simulink model "ECS_FOS"  (R2013b)
settings: Solver=ode45  StartTime=0.0  StopTime=10.0  RelTol=1e-3
values from neighbouring files (symbols this model uses):
  FuelBurn = [0 0 0 0 0 0 0 0 0 0 0 0 ... (18249 elements, 1x18249)]    [Benchmark_data1.mat]
undefined symbols (not defined in the file or in its folder): F1, F2, HUGHES_TREITLER, PN_70147
libraries: PowerFlowLib x47, simulink x6
(part 1 of 2)
settings Model: Creator=mwillms4  LastModifiedBy=mwillms4

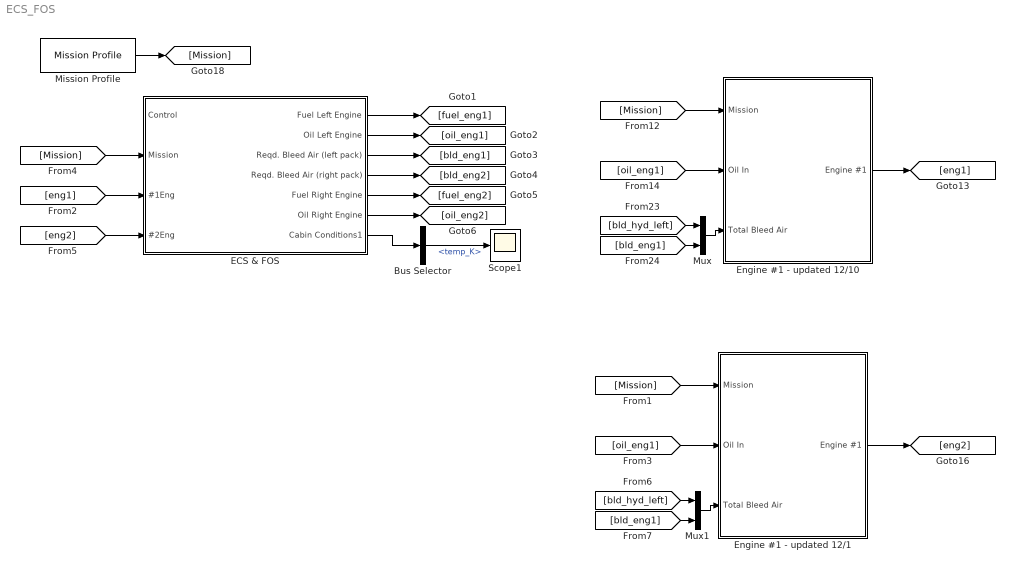
== system ECS_FOS ==
  Bus Selector : BusSelector  OutputSignals=temp_K
  "ECS & FOS " : Subsystem
  Engine #1 - updated 12/1 : Subsystem
  Engine #1 - updated 12/10 : Subsystem
  Mission Profile : PowerFlowLib/Mission Profile/Mission Profile  mssn_check=off  mssn_prof=MSSN  del_P=0  del_T=0  del_rho=0  pres_msl=101.3  temp_msl=15  dens_msl=1.229
  Mux : Mux  Inputs=2
  Mux1 : Mux  Inputs=2
  Scope1 : Scope
      settings: YMin=290  YMax=300
  wires:
  Mission Profile/1 -> [Mission]
  [eng1] -> "ECS & FOS "/3(#1Eng)
  [Mission] -> "ECS & FOS "/2(Mission)
  [eng2] -> "ECS & FOS "/4(#2Eng)
  Engine #1 - updated 12/10/1(Engine #1) -> [eng1]
  Engine #1 - updated 12/1/1(Engine #1) -> [eng2]
  [Mission] -> Engine #1 - updated 12/10/1(Mission)
  [oil_eng1] -> Engine #1 - updated 12/10/2(Oil In)
  Mux/1 -> Engine #1 - updated 12/10/3(Total Bleed Air)
  [bld_eng1] -> Mux/2
  [bld_hyd_left] -> Mux/1
  Bus Selector/1 -> Scope1/1  "<temp_K>"
  "ECS & FOS "/1("Fuel Left Engine ") -> [fuel_eng1]
  "ECS & FOS "/2(Oil Left Engine) -> [oil_eng1]
  "ECS & FOS "/3(Reqd. Bleed Air (left pack)) -> [bld_eng1]
  "ECS & FOS "/4(Reqd. Bleed Air (right pack)) -> [bld_eng2]
  "ECS & FOS "/5(Fuel Right Engine) -> [fuel_eng2]
  "ECS & FOS "/6(Oil Right Engine) -> [oil_eng2]
  "ECS & FOS "/7(Cabin Conditions1) -> Bus Selector/1
  [Mission] -> Engine #1 - updated 12/1/1(Mission)
  [oil_eng1] -> Engine #1 - updated 12/1/2(Oil In)
  Mux1/1 -> Engine #1 - updated 12/1/3(Total Bleed Air)
  [bld_eng1] -> Mux1/2
  [bld_hyd_left] -> Mux1/1

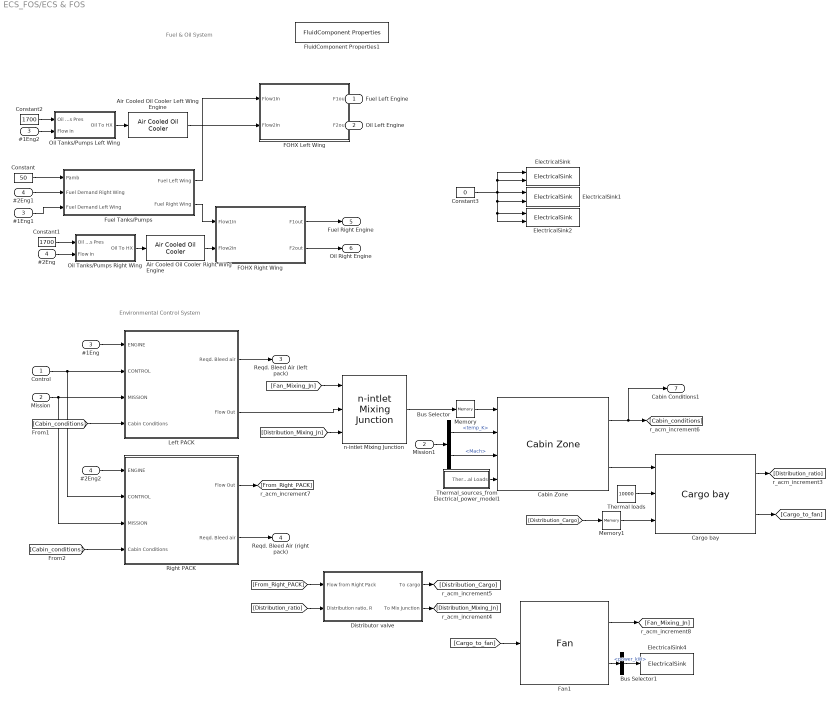
== system ECS_FOS/ECS & FOS  ==
  note: Fuel & Oil System
  note: Environmental Control System
  Control : Inport
  Mission : Inport  Port=2
  #1Eng : Inport  Port=3
  #2Eng : Inport  Port=4
  #1Eng1 : InportShadow  Port=3
  #1Eng2 : InportShadow  Port=3
  #2Eng1 : InportShadow  Port=4
  #2Eng2 : InportShadow  Port=4
  Air Cooled Oil Cooler Left Wing Engine : PowerFlowLib/Energy & Power Systems/Thermal/Oil/Air Cooled Oil Cooler  fileslct=off  filename=HeatExchangers.mat  filedir=C:\Users\mwillms4\Dropbox\School\Graduate\Research\PowerFlow Summer 2013\PropertyTables\HeatExchangers.mat  refresh=off  hx=HUGHES_TREITLER - PN_70147  bypass_full=1  bypass_none=100  hx_delP=82.74  hx_P=2068  hx_Qdot=24.27  hx_Vdot=0.000505  hx_mass=4.42
  Air Cooled Oil Cooler Right Wing Engine : PowerFlowLib/Energy & Power Systems/Thermal/Oil/Air Cooled Oil Cooler  fileslct=off  filename=HeatExchangers.mat  filedir=C:\Users\mwillms4\Dropbox\School\Graduate\Research\PowerFlow Summer 2013\PropertyTables\HeatExchangers.mat  refresh=off  hx=HUGHES_TREITLER - PN_70147  bypass_full=1  bypass_none=100  hx_delP=82.74  hx_P=2068  hx_Qdot=24.27  hx_Vdot=0.000505  hx_mass=4.42
  Bus Selector : BusSelector  OutputSignals=Flight parameters.temp_K,Flight parameters.Mach
  Bus Selector1 : BusSelector  OutputSignals=power_kW
  Cabin Zone : PowerFlowLib/Energy & Power Systems/Thermal/ECS/Cabin Zone  A_fuselage=320  V_cab=130.3  n_pass=176  L_shell=0.003  K_shell=1  L_insulation=0.02  K_insulation=1  L_coating=0.002  K_coating=1  Vdot_sa_pass=0.009438  q_pass=60  RAR=.25  h_outside=1  h_inside=1
  Cargo bay : PowerFlowLib/Energy & Power Systems/Thermal/ECS/Cargo bay  T_cargo_K=305
  Constant : Constant  Value=50
  Constant1 : Constant  Value=1700
  Constant2 : Constant  Value=1700
  Constant3 : Constant  Value=0
  Distributor valve : Subsystem
  ElectricalSink : PowerFlowLib/Support Functions//Tools/ElectricalSink  Tag=Flow  Description=TwoPhase  load_loc=Empennage  ACDC_load=AC  units=Kilowatts  unq_id=9254
  ElectricalSink1 : PowerFlowLib/Support Functions//Tools/ElectricalSink  Tag=Flow  Description=TwoPhase  load_loc=Cagobay  ACDC_load=AC  units=Kilowatts  unq_id=3572
  ElectricalSink2 : PowerFlowLib/Support Functions//Tools/ElectricalSink  Tag=Flow  Description=TwoPhase  load_loc=Cabin  ACDC_load=AC  units=Kilowatts  unq_id=7814
  ElectricalSink4 : PowerFlowLib/Support Functions//Tools/ElectricalSink  Tag=Flow  Description=TwoPhase  load_loc=Cabin  ACDC_load=DC  units=Kilowatts  unq_id=7783
  FOHX Left Wing : Subsystem  Description=TwoPhase  mask{fld1=JP8, fld2=LubeOil7808, alpha1=80, alpha2=80, N1=10, N2=10, A1_c=.1, A2_c=.1, A1_s=.25, A2_s=.25, P1init=620.5, P2init=620.5}
      mask prompts: fld1 "Fluid 1 Type"; fld2 "Fluid 2 Type"; alpha1 "Fluid 1 HTC [W/m² K]"; alpha2 "Fluid 2 HTC [W/m² K]"; N1 "Flow 1: Number of Channels"; N2 "Flow 2: Number of Channels"; A1_c "Flow 1: Cross-sectional area [m^2]"; A2_c "Flow 2: Cross-sectional area [m^2]"; A1_s "Flow 1: Total surface area [m^2]"; A2_s "Flow 2: Total surface area [m^2]"; P1init "Flow 1 Pressure [kPa]"; P2init "Flow 2 Pressure [kPa]"
      mask init:
      | %load TMSFluidProperties
      | %eval(['SF = FluidProp.SinglePhase.' get_param(gcb,'fld_type1') ';']);
      | %eval(['F = FluidProp.TwoPhase.' get_param(gcb,'fld_type2') ';']);
      | %FluidProp = FluidProp.TwoPhase.R134a; 
      | %{
      | if strcmp(get_param(bdroot,'SimulationStatus'),'initializing') ;
      |     load TwoPhaseProp_Evap
      |     TwoPhaseProp = TwoPhaseProp_Evap;
      |     Evaporator_Init_AFRL;
      | end
      | TMS_SetPhysSigs
      | if strcmp(get_param(gcb,'fld_type1'),'MoistAir')
      |     notair = 0 ; 
      | else
      |     notair = 1 ;
      | end
      | %}
      mask TypeOptions fld1: JP8
      mask TypeOptions fld2: LubeOil7808
      mask Display:
      | port_label('input',1,'Fuel In','TexMode','on') ;
      | port_label('input',2,'Oil In','TexMode','on') ;
      | port_label('output',1,'Fuel Out','TexMode','on') ;
      | port_label('output',2,'Oil Out','TexMode','on') ;
  FOHX Right Wing : Subsystem  Description=TwoPhase  mask{fld1=JP8, fld2=LubeOil7808, alpha1=80, alpha2=80, N1=10, N2=10, A1_c=.1, A2_c=.1, A1_s=.25, A2_s=.25, P1init=620.5, P2init=620.5}
      mask prompts: fld1 "Fluid 1 Type"; fld2 "Fluid 2 Type"; alpha1 "Fluid 1 HTC [W/m² K]"; alpha2 "Fluid 2 HTC [W/m² K]"; N1 "Flow 1: Number of Channels"; N2 "Flow 2: Number of Channels"; A1_c "Flow 1: Cross-sectional area [m^2]"; A2_c "Flow 2: Cross-sectional area [m^2]"; A1_s "Flow 1: Total surface area [m^2]"; A2_s "Flow 2: Total surface area [m^2]"; P1init "Flow 1 Pressure [kPa]"; P2init "Flow 2 Pressure [kPa]"
      mask init: same as ECS_FOS/ECS & FOS /FOHX Left Wing
      mask TypeOptions fld1: JP8
      mask TypeOptions fld2: LubeOil7808
      mask Display:
      | port_label('input',1,'Fuel In','TexMode','on') ;
      | port_label('input',2,'Oil In','TexMode','on') ;
      | port_label('output',1,'Fuel Out','TexMode','on') ;
      | port_label('output',2,'Oil Out','TexMode','on') ;
  Fan1 : PowerFlowLib/Energy & Power Systems/Thermal/ECS/Fan  N_fan=1725
  FluidComponent Properties1 : PowerFlowLib/Support Functions//Tools/FluidComponent Properties  fuelprop=FluidProp_JetA3638.mat  oilprop=OilProp.mat  airprop=AirProp.mat  pumpprop=PumpProp.mat  fanprop=Fanmap.mat  compprop=CompProp.mat  heatexprop=HeatExchangers.mat
  Fuel Tanks/Pumps : Subsystem
  Left PACK : Subsystem
  Memory : Memory
  Memory1 : Memory
  Mission1 : InportShadow  Port=2
  Oil Tanks/Pumps Left Wing : Subsystem
  Oil Tanks/Pumps Right Wing : Subsystem
  Right PACK : Subsystem
  Thermal loads : Constant  Value=10000
  Thermal_sources_from Electrical_power_model1 : Subsystem
  n-intlet Mixing Junction : PowerFlowLib/Energy & Power Systems/Thermal/ECS/n-intlet Mixing Junction  no_inlets=3  d_in_1=0.1  d_in_2=0.1  d_out=0.2
  "Fuel Left Engine " : Outport
  Oil Left Engine : Outport  Port=2
  Reqd. Bleed Air (left pack) : Outport  Port=3
  Reqd. Bleed Air (right pack) : Outport  Port=4
  Fuel Right Engine : Outport  Port=5
  Oil Right Engine : Outport  Port=6
  Cabin Conditions1 : Outport  Port=7
  wires:
  Cargo bay/2 -> [Cargo_to_fan]
  Cabin Zone/2 -> Cargo bay/1
  Memory1/1 -> Cargo bay/3
  Thermal loads/1 -> Cargo bay/2
  Cargo bay/1 -> [Distribution_ratio]
  [Distribution_Cargo] -> Memory1/1
  Fan1/2 -> Bus Selector1/1
  Fan1/1 -> [Fan_Mixing_Jn]
  [Cargo_to_fan] -> Fan1/1
  Bus Selector1/1 -> ElectricalSink4/1  "<power_kW>"
  [Distribution_Mixing_Jn] -> n-intlet Mixing Junction/3
  Right PACK/1(Flow Out) -> [From_Right_PACK]
  [Cabin_conditions] -> Left PACK/4(Cabin Conditions)
  [Cabin_conditions] -> Right PACK/4(Cabin Conditions)
  [Fan_Mixing_Jn] -> n-intlet Mixing Junction/1
  Cabin Zone/1 -> [Cabin_conditions], Cabin Conditions1/1
  Distributor valve/1(To cargo) -> [Distribution_Cargo]
  Distributor valve/2(To Mix Junction) -> [Distribution_Mixing_Jn]
  [From_Right_PACK] -> Distributor valve/1(Flow from Right Pack)
  [Distribution_ratio] -> Distributor valve/2("Distribution ratio, R")
  #2Eng2/1 -> Right PACK/1(ENGINE)
  #1Eng/1 -> Left PACK/1(ENGINE)
  #2Eng/1 -> Oil Tanks/Pumps Right Wing/2(Flow In)
  #1Eng1/1 -> Fuel Tanks/Pumps/3(Fuel Demand Left Wing)
  #2Eng1/1 -> Fuel Tanks/Pumps/2(Fuel Demand Right Wing)
  #1Eng2/1 -> Oil Tanks/Pumps Left Wing/2(Flow In)
  Memory/1 -> Cabin Zone/1
  Left PACK/2(Flow Out) -> n-intlet Mixing Junction/2
  Thermal_sources_from Electrical_power_model1/1(Thermal Loads) -> Cabin Zone/4
  Bus Selector/2 -> Cabin Zone/3  "<Mach>"
  Bus Selector/1 -> Cabin Zone/2  "<temp_K>"
  Mission1/1 -> Bus Selector/1
  n-intlet Mixing Junction/1 -> Memory/1
  Constant3/1 -> ElectricalSink/2, ElectricalSink/1, ElectricalSink1/2, ElectricalSink2/2, ElectricalSink2/1, ElectricalSink1/1
  FOHX Left Wing/2(F2out) -> Oil Left Engine/1
  FOHX Right Wing/2(F2out) -> Oil Right Engine/1
  FOHX Left Wing/1(F1out) -> "Fuel Left Engine "/1
  Fuel Tanks/Pumps/1(Fuel Left Wing) -> FOHX Left Wing/1(Flow1In)
  Constant2/1 -> Oil Tanks/Pumps Left Wing/1(Oil Sys Pres)
  Oil Tanks/Pumps Left Wing/1(Oil To HX) -> Air Cooled Oil Cooler Left Wing Engine/1
  Air Cooled Oil Cooler Left Wing Engine/1 -> FOHX Left Wing/2(Flow2In)
  FOHX Right Wing/1(F1out) -> Fuel Right Engine/1
  Constant1/1 -> Oil Tanks/Pumps Right Wing/1(Oil Sys Pres)
  Oil Tanks/Pumps Right Wing/1(Oil To HX) -> Air Cooled Oil Cooler Right Wing Engine/1
  Fuel Tanks/Pumps/2(Fuel Right Wing) -> FOHX Right Wing/1(Flow1In)
  Air Cooled Oil Cooler Right Wing Engine/1 -> FOHX Right Wing/2(Flow2In)
  Constant/1 -> Fuel Tanks/Pumps/1(Pamb)
  Right PACK/2(Reqd. Bleed air) -> Reqd. Bleed Air (right pack)/1
  Mission/1 -> Right PACK/3(MISSION), Left PACK/3(MISSION)
  Control/1 -> Right PACK/2(CONTROL), Left PACK/2(CONTROL)
  Left PACK/1(Reqd. Bleed air) -> Reqd. Bleed Air (left pack)/1

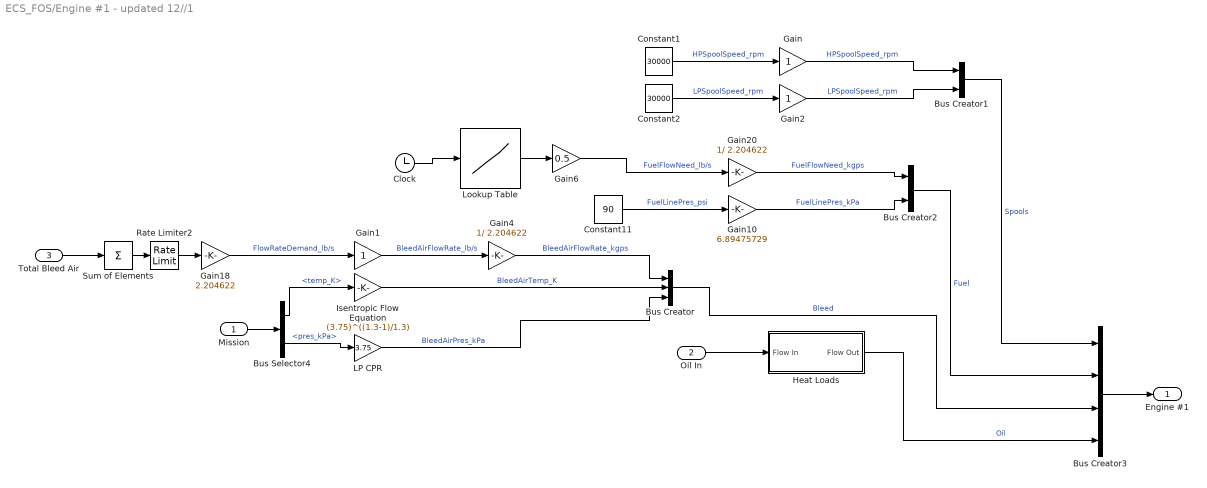
== system ECS_FOS/Engine #1 - updated 12//1 ==
  Mission : Inport
  Oil In : Inport  Port=2
  Total Bleed Air : Inport  Port=3
  Bus Creator : BusCreator  Inputs=3
  Bus Creator1 : BusCreator  Inputs=2
  Bus Creator2 : BusCreator  Inputs=2
  Bus Creator3 : BusCreator
  Bus Selector4 : BusSelector  OutputSignals=Flight parameters.temp_K,Flight parameters.pres_kPa
  Clock : Clock
  Constant1 : Constant  Value=30000
  Constant11 : Constant  Value=90
  Constant2 : Constant  Value=30000
  Gain : Gain
  Gain1 : Gain
  Gain10 : Gain  Gain=6.89475729
  Gain18 : Gain  Gain=2.204622
  Gain2 : Gain
  Gain20 : Gain  Gain=1/ 2.204622
  Gain4 : Gain  Gain=1/ 2.204622
  Gain6 : Gain  Gain=0.5
  Heat Loads : Subsystem
  Isentropic Flow Equation : Gain  Gain=(3.75)^((1.3-1)/1.3)
  LP CPR : Gain  Gain=3.75
  Lookup Table : Lookup  InputValues=[0:size(FuelBurn,2)-1]  Table=FuelBurn
  Rate Limiter2 : RateLimiter
  Sum of Elements : Sum  Inputs=+
  Engine #1 : Outport
  wires:
  Bus Creator3/1 -> Engine #1/1
  Lookup Table/1 -> Gain6/1
  Clock/1 -> Lookup Table/1
  Bus Selector4/1 -> Isentropic Flow Equation/1  "<temp_K>"
  Bus Selector4/2 -> LP CPR/1  "<pres_kPa>"
  Mission/1 -> Bus Selector4/1
  Sum of Elements/1 -> Rate Limiter2/1
  Bus Creator2/1 -> Bus Creator3/2  "Fuel"
  Bus Creator1/1 -> Bus Creator3/1  "Spools"
  Bus Creator/1 -> Bus Creator3/3  "Bleed"
  Heat Loads/1(Flow Out) -> Bus Creator3/4  "Oil"
  Oil In/1 -> Heat Loads/1(Flow In)
  Rate Limiter2/1 -> Gain18/1
  Gain18/1 -> Gain1/1  "FlowRateDemand_lb/s"
  Total Bleed Air/1 -> Sum of Elements/1
  Gain/1 -> Bus Creator1/1  "HPSpoolSpeed_rpm"
  Constant1/1 -> Gain/1  "HPSpoolSpeed_rpm"
  Gain2/1 -> Bus Creator1/2  "LPSpoolSpeed_rpm"
  Constant2/1 -> Gain2/1  "LPSpoolSpeed_rpm"
  Gain4/1 -> Bus Creator/1  "BleedAirFlowRate_kgps"
  Gain1/1 -> Gain4/1  "BleedAirFlowRate_lb/s"
  Isentropic Flow Equation/1 -> Bus Creator/2  "BleedAirTemp_K"
  LP CPR/1 -> Bus Creator/3  "BleedAirPres_kPa"
  Gain20/1 -> Bus Creator2/1  "FuelFlowNeed_kgps"
  Gain6/1 -> Gain20/1  "FuelFlowNeed_lb/s"
  Gain10/1 -> Bus Creator2/2  "FuelLinePres_kPa"
  Constant11/1 -> Gain10/1  "FuelLinePres_psi"

== system ECS_FOS/Engine #1 - updated 12//10 ==
  Mission : Inport
  Oil In : Inport  Port=2
  Total Bleed Air : Inport  Port=3
  Bus Creator : BusCreator  Inputs=3
  Bus Creator1 : BusCreator  Inputs=2
  Bus Creator2 : BusCreator  Inputs=2
  Bus Creator3 : BusCreator
  Bus Selector4 : BusSelector  OutputSignals=Flight parameters.temp_K,Flight parameters.pres_kPa
  Clock : Clock
  Constant1 : Constant  Value=30000
  Constant11 : Constant  Value=90
  Constant2 : Constant  Value=30000
  Gain : Gain
  Gain1 : Gain
  Gain10 : Gain  Gain=6.89475729
  Gain18 : Gain  Gain=2.204622
  Gain2 : Gain
  Gain20 : Gain  Gain=1/ 2.204622
  Gain4 : Gain  Gain=1/ 2.204622
  Gain6 : Gain  Gain=0.5
  Heat Loads : Subsystem
  Isentropic Flow Equation : Gain  Gain=(3.75)^((1.3-1)/1.3)
  LP CPR : Gain  Gain=3.75
  Lookup Table : Lookup  InputValues=[0:size(FuelBurn,2)-1]  Table=FuelBurn
  Rate Limiter2 : RateLimiter
  Sum of Elements : Sum  Inputs=+
  Engine #1 : Outport
  wires:
  Constant11/1 -> Gain10/1  "FuelLinePres_psi"
  Gain10/1 -> Bus Creator2/2  "FuelLinePres_kPa"
  Gain6/1 -> Gain20/1  "FuelFlowNeed_lb/s"
  Gain20/1 -> Bus Creator2/1  "FuelFlowNeed_kgps"
  LP CPR/1 -> Bus Creator/3  "BleedAirPres_kPa"
  Isentropic Flow Equation/1 -> Bus Creator/2  "BleedAirTemp_K"
  Gain1/1 -> Gain4/1  "BleedAirFlowRate_lb/s"
  Gain4/1 -> Bus Creator/1  "BleedAirFlowRate_kgps"
  Constant2/1 -> Gain2/1  "LPSpoolSpeed_rpm"
  Gain2/1 -> Bus Creator1/2  "LPSpoolSpeed_rpm"
  Constant1/1 -> Gain/1  "HPSpoolSpeed_rpm"
  Gain/1 -> Bus Creator1/1  "HPSpoolSpeed_rpm"
  Total Bleed Air/1 -> Sum of Elements/1
  Gain18/1 -> Gain1/1  "FlowRateDemand_lb/s"
  Rate Limiter2/1 -> Gain18/1
  Oil In/1 -> Heat Loads/1(Flow In)
  Heat Loads/1(Flow Out) -> Bus Creator3/4  "Oil"
  Bus Creator/1 -> Bus Creator3/3  "Bleed"
  Bus Creator1/1 -> Bus Creator3/1  "Spools"
  Bus Creator2/1 -> Bus Creator3/2  "Fuel"
  Sum of Elements/1 -> Rate Limiter2/1
  Mission/1 -> Bus Selector4/1
  Bus Selector4/2 -> LP CPR/1  "<pres_kPa>"
  Bus Selector4/1 -> Isentropic Flow Equation/1  "<temp_K>"
  Clock/1 -> Lookup Table/1
  Lookup Table/1 -> Gain6/1
  Bus Creator3/1 -> Engine #1/1

== system ECS_FOS/ECS & FOS /Distributor valve ==
  Flow from Right Pack : Inport
  "Distribution ratio, R" : Inport  Port=2
  Bus Creator : BusCreator  Inputs=3
  Bus Creator1 : BusCreator  Inputs=3
  Bus Selector1 : BusSelector  OutputSignals=mdot_kgps,temp_K,pres_kPa
  M(1-R) : Sum  Inputs=+-
  Product : Product
  To cargo : Outport
  To Mix Junction : Outport  Port=2
  wires:
  Bus Selector1/3 -> Bus Creator1/3, Bus Creator/3  "<pres_kPa>"
  Bus Selector1/2 -> Bus Creator1/2, Bus Creator/2  "<temp_K>"
  Bus Creator1/1 -> To cargo/1
  Bus Creator/1 -> To Mix Junction/1
  M(1-R)/1 -> Bus Creator/1  "mdot_kgps"
  Product/1 -> M(1-R)/2, Bus Creator1/1  "mdot_kgps"
  "Distribution ratio, R"/1 -> Product/2
  Bus Selector1/1 -> Product/1, M(1-R)/1  "<mdot_kgps>"
  Flow from Right Pack/1 -> Bus Selector1/1

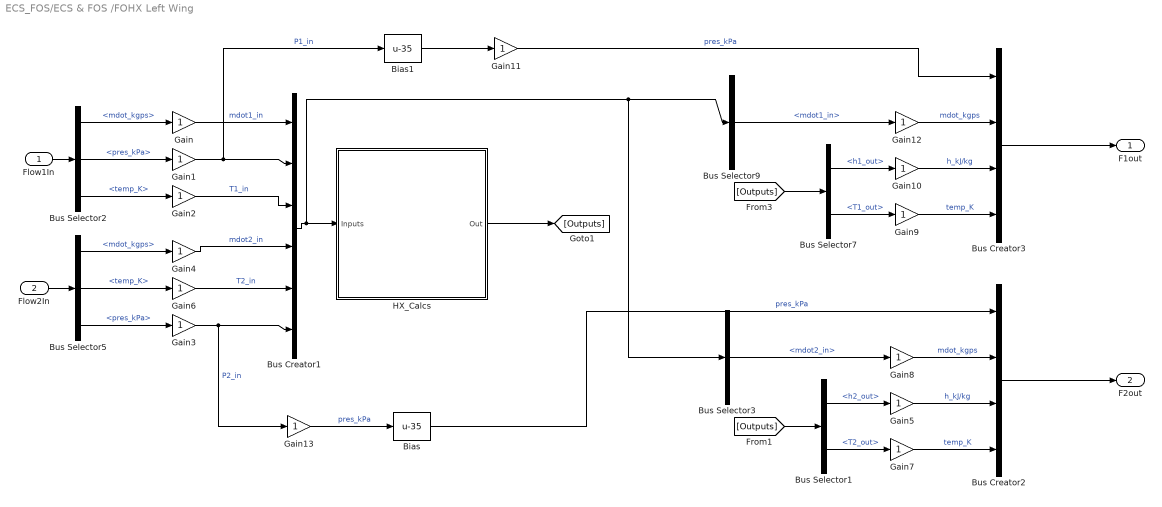
== system ECS_FOS/ECS & FOS /FOHX Left Wing ==
  Flow1In : Inport
  Flow2In : Inport  Port=2
  Bias : Bias  Bias=-35
  Bias1 : Bias  Bias=-35
  Bus Creator1 : BusCreator  Inputs=6
  Bus Creator2 : BusCreator
  Bus Creator3 : BusCreator
  Bus Selector1 : BusSelector  OutputSignals=h2_out,T2_out
  Bus Selector2 : BusSelector  OutputSignals=mdot_kgps,pres_kPa,temp_K
  Bus Selector3 : BusSelector  OutputSignals=mdot2_in
  Bus Selector5 : BusSelector  OutputSignals=mdot_kgps,temp_K,pres_kPa
  Bus Selector7 : BusSelector  OutputSignals=h1_out,T1_out
  Bus Selector9 : BusSelector  OutputSignals=mdot1_in
  Gain{,1..13} (14 alike) : Gain
  HX_Calcs : Subsystem
  F1out : Outport
  F2out : Outport  Port=2
  wires:
  Bus Selector7/2 -> Gain9/1  "<T1_out>"
  Bus Selector7/1 -> Gain10/1  "<h1_out>"
  Bus Selector9/1 -> Gain12/1  "<mdot1_in>"
  [Outputs] -> Bus Selector7/1
  Gain9/1 -> Bus Creator3/4  "temp_K"
  Gain10/1 -> Bus Creator3/3  "h_kJ/kg"
  Gain12/1 -> Bus Creator3/2  "mdot_kgps"
  Bus Creator3/1 -> F1out/1
  Bus Creator2/1 -> F2out/1
  Bus Selector5/1 -> Gain4/1  "<mdot_kgps>"
  Bus Selector5/2 -> Gain6/1  "<temp_K>"
  Flow2In/1 -> Bus Selector5/1
  Bus Selector2/3 -> Gain2/1  "<temp_K>"
  Bus Selector2/2 -> Gain1/1  "<pres_kPa>"
  Bus Selector2/1 -> Gain/1  "<mdot_kgps>"
  Bus Creator1/1 -> HX_Calcs/1(Inputs), Bus Selector9/1, Bus Selector3/1
  Flow1In/1 -> Bus Selector2/1
  HX_Calcs/1(Out) -> [Outputs]
  Gain6/1 -> Bus Creator1/5  "T2_in"
  Gain4/1 -> Bus Creator1/4  "mdot2_in"
  Gain2/1 -> Bus Creator1/3  "T1_in"
  Gain1/1 -> Bus Creator1/2, Bias1/1  "P1_in"
  Gain/1 -> Bus Creator1/1  "mdot1_in"
  Bus Selector5/3 -> Gain3/1  "<pres_kPa>"
  Gain3/1 -> Bus Creator1/6, Gain13/1  "P2_in"
  Bus Selector1/2 -> Gain7/1  "<T2_out>"
  Bus Selector1/1 -> Gain5/1  "<h2_out>"
  [Outputs] -> Bus Selector1/1
  Gain7/1 -> Bus Creator2/4  "temp_K"
  Gain5/1 -> Bus Creator2/3  "h_kJ/kg"
  Bus Selector3/1 -> Gain8/1  "<mdot2_in>"
  Gain8/1 -> Bus Creator2/2  "mdot_kgps"
  Gain11/1 -> Bus Creator3/1  "pres_kPa"
  Gain13/1 -> Bias/1  "pres_kPa"
  Bias/1 -> Bus Creator2/1  "pres_kPa"
  Bias1/1 -> Gain11/1

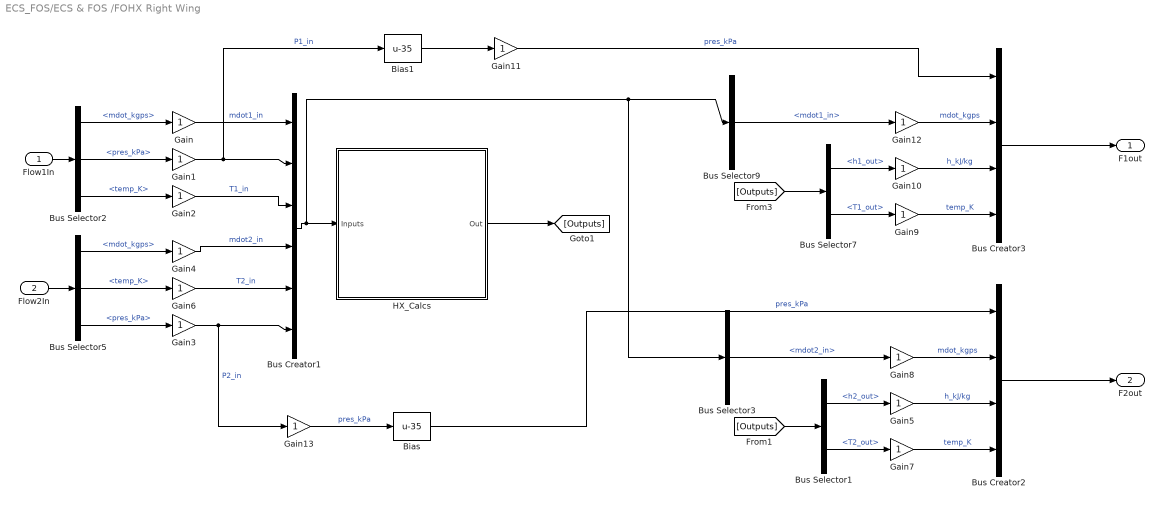
== system ECS_FOS/ECS & FOS /FOHX Right Wing ==
  Flow1In : Inport
  Flow2In : Inport  Port=2
  Bias : Bias  Bias=-35
  Bias1 : Bias  Bias=-35
  Bus Creator1 : BusCreator  Inputs=6
  Bus Creator2 : BusCreator
  Bus Creator3 : BusCreator
  Bus Selector1 : BusSelector  OutputSignals=h2_out,T2_out
  Bus Selector2 : BusSelector  OutputSignals=mdot_kgps,pres_kPa,temp_K
  Bus Selector3 : BusSelector  OutputSignals=mdot2_in
  Bus Selector5 : BusSelector  OutputSignals=mdot_kgps,temp_K,pres_kPa
  Bus Selector7 : BusSelector  OutputSignals=h1_out,T1_out
  Bus Selector9 : BusSelector  OutputSignals=mdot1_in
  Gain{,1..13} (14 alike) : Gain
  HX_Calcs : Subsystem
  F1out : Outport
  F2out : Outport  Port=2
  wires:
  Bias1/1 -> Gain11/1
  Bias/1 -> Bus Creator2/1  "pres_kPa"
  Gain13/1 -> Bias/1  "pres_kPa"
  Gain11/1 -> Bus Creator3/1  "pres_kPa"
  Gain8/1 -> Bus Creator2/2  "mdot_kgps"
  Bus Selector3/1 -> Gain8/1  "<mdot2_in>"
  Gain5/1 -> Bus Creator2/3  "h_kJ/kg"
  Gain7/1 -> Bus Creator2/4  "temp_K"
  [Outputs] -> Bus Selector1/1
  Bus Selector1/1 -> Gain5/1  "<h2_out>"
  Bus Selector1/2 -> Gain7/1  "<T2_out>"
  Gain3/1 -> Gain13/1, Bus Creator1/6  "P2_in"
  Bus Selector5/3 -> Gain3/1  "<pres_kPa>"
  Gain/1 -> Bus Creator1/1  "mdot1_in"
  Gain1/1 -> Bias1/1, Bus Creator1/2  "P1_in"
  Gain2/1 -> Bus Creator1/3  "T1_in"
  Gain4/1 -> Bus Creator1/4  "mdot2_in"
  Gain6/1 -> Bus Creator1/5  "T2_in"
  HX_Calcs/1(Out) -> [Outputs]
  Flow1In/1 -> Bus Selector2/1
  Bus Creator1/1 -> Bus Selector3/1, Bus Selector9/1, HX_Calcs/1(Inputs)
  Bus Selector2/1 -> Gain/1  "<mdot_kgps>"
  Bus Selector2/2 -> Gain1/1  "<pres_kPa>"
  Bus Selector2/3 -> Gain2/1  "<temp_K>"
  Flow2In/1 -> Bus Selector5/1
  Bus Selector5/2 -> Gain6/1  "<temp_K>"
  Bus Selector5/1 -> Gain4/1  "<mdot_kgps>"
  Bus Creator2/1 -> F2out/1
  Bus Creator3/1 -> F1out/1
  Gain12/1 -> Bus Creator3/2  "mdot_kgps"
  Gain10/1 -> Bus Creator3/3  "h_kJ/kg"
  Gain9/1 -> Bus Creator3/4  "temp_K"
  [Outputs] -> Bus Selector7/1
  Bus Selector9/1 -> Gain12/1  "<mdot1_in>"
  Bus Selector7/1 -> Gain10/1  "<h1_out>"
  Bus Selector7/2 -> Gain9/1  "<T1_out>"

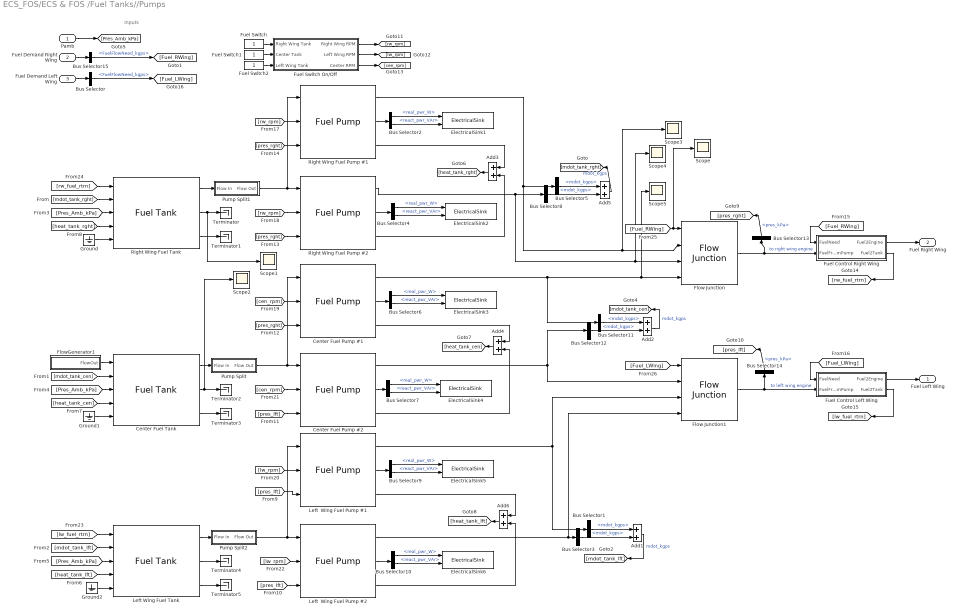
== system ECS_FOS/ECS & FOS /Fuel Tanks//Pumps ==
  note: Inputs
  Pamb : Inport
  Fuel Demand Right Wing : Inport  Port=2
  Fuel Demand Left Wing : Inport  Port=3
  Add{1..6} (6 alike) : Sum
  Bus Selector : BusSelector  OutputSignals=Fuel.FuelFlowNeed_kgps
  Bus Selector{1,3,5,8,11..12} (6 alike) : BusSelector  OutputSignals=mdot_kgps
  Bus Selector{2,4,6..7,9..10} (6 alike) : BusSelector  OutputSignals=real_pwr_W,react_pwr_VAr
  Bus Selector13 : BusSelector  OutputSignals=pres_kPa
  Bus Selector14 : BusSelector  OutputSignals=pres_kPa
  Bus Selector15 : BusSelector  OutputSignals=Fuel.FuelFlowNeed_kgps
  Center Fuel Pump #1 : PowerFlowLib/Energy & Power Systems/Thermal/Fuel/Fuel Pump  maptype=Pressure (kPa) vs. Vol. Flow Rate (m³/hr)  map=B737_AC_fuel1  map_load=off  SG=0.82  pump_eff=.75  heat_out=off  AC_pwr=on  pf=1  mech_pwr=off
  Center Fuel Pump #2 : PowerFlowLib/Energy & Power Systems/Thermal/Fuel/Fuel Pump  maptype=Pressure (kPa) vs. Vol. Flow Rate (m³/hr)  map=B737_AC_fuel1  map_load=off  SG=0.82  pump_eff=.75  heat_out=off  AC_pwr=on  pf=1  mech_pwr=off
  Center Fuel Tank : PowerFlowLib/Energy & Power Systems/Thermal/Fuel/Fuel Tank  fileslct=off  filename=fueltank_area.m  filedir=C:\Users\mwillms4\Documents\My Box Files\Graduate\Research\PowerFlow Development\PowerFlow Fall 2013\SupportFunctions\fueltank_area.m  tank_loc=Center Tank  areaprompt2=off  max_vol=3.2  m_init=2500  fld_Tint=0  ull_Tint=30  Pover=100  HTC_fg=14.2  wallHXF=off  wetHTC=14.2  dryHTC=14.2  Qinternal=0
  ElectricalSink1 : PowerFlowLib/Support Functions//Tools/ElectricalSink  Tag=Flow  Description=TwoPhase  load_loc=RightWing  ACDC_load=AC  units=Watts  unq_id=4424
  ElectricalSink2 : PowerFlowLib/Support Functions//Tools/ElectricalSink  Tag=Flow  Description=TwoPhase  load_loc=RightWing  ACDC_load=AC  units=Watts  unq_id=6110
  ElectricalSink3 : PowerFlowLib/Support Functions//Tools/ElectricalSink  Tag=Flow  Description=TwoPhase  load_loc=RightWing  ACDC_load=AC  units=Watts  unq_id=1683
  ElectricalSink4 : PowerFlowLib/Support Functions//Tools/ElectricalSink  Tag=Flow  Description=TwoPhase  load_loc=LeftWing  ACDC_load=AC  units=Watts  unq_id=1485
  ElectricalSink5 : PowerFlowLib/Support Functions//Tools/ElectricalSink  Tag=Flow  Description=TwoPhase  load_loc=LeftWing  ACDC_load=AC  units=Watts  unq_id=5777
  ElectricalSink6 : PowerFlowLib/Support Functions//Tools/ElectricalSink  Tag=Flow  Description=TwoPhase  load_loc=LeftWing  ACDC_load=AC  units=Watts  unq_id=8012
  Flow Junction : PowerFlowLib/Energy & Power Systems/Thermal/Fuel/Flow Junction  Description=TwoPhase  V=.05  Bm=10^5  initPres=6000  initTemp=30
  Flow Junction1 : PowerFlowLib/Energy & Power Systems/Thermal/Fuel/Flow Junction  Description=TwoPhase  V=.05  Bm=10^5  initPres=6000  initTemp=30
  FlowGenerator1 : Subsystem  Tag=Flow  Description=TwoPhase  mask{fld_type1=null, flowrate=0, flowtemp=0, flowpres=00, flowenthalpy=0}
      mask prompts: fld_type1 "Fluid Type"; flowrate "Fluid Flow Rate (kg/s)"; flowtemp "Fluid Flow Temperature (C)"; flowpres "Fluid Flow Pressure (kPa)"; flowenthalpy "Fluid Flow Enthalpy (kJ/kg)"
      mask TypeOptions fld_type1: null
      mask Display: text(.5,.5,'Flow Source','horizontalAlignment','center','texmode','on')
  Fuel Control Left Wing : Subsystem
      mask Display:
      | port_label('input',1,'{\bf Fuel Need}','TexMode','on')
      | port_label('input',2,'{\bf Fuel In}','TexMode','on')
      | 
      | 
      | port_label('output',1,'{\bf Fuel to Eng.}','TexMode','on')
      | port_label('output',2,'{\bf Fuel Return}','TexMode','on')
  "Fuel Control Right Wing " : Subsystem
      mask Display:
      | port_label('input',1,'{\bf Fuel Need}','TexMode','on')
      | port_label('input',2,'{\bf Fuel In}','TexMode','on')
      | 
      | 
      | port_label('output',1,'{\bf Fuel to Eng.}','TexMode','on')
      | port_label('output',2,'{\bf Fuel Return}','TexMode','on')
  Fuel Switch : Constant
  Fuel Switch On/Off : Subsystem
  Fuel Switch1 : Constant
  Fuel Switch2 : Constant
  Ground : Ground
  Ground1 : Ground
  Ground2 : Ground
  Left  Wing Fuel Pump #1 : PowerFlowLib/Energy & Power Systems/Thermal/Fuel/Fuel Pump  maptype=Pressure (kPa) vs. Vol. Flow Rate (m³/hr)  map=B737_AC_fuel1  map_load=off  SG=0.82  pump_eff=.75  heat_out=off  AC_pwr=on  pf=1  mech_pwr=off
  Left  Wing Fuel Pump #2 : PowerFlowLib/Energy & Power Systems/Thermal/Fuel/Fuel Pump  maptype=Pressure (kPa) vs. Vol. Flow Rate (m³/hr)  map=B737_AC_fuel1  map_load=off  SG=0.82  pump_eff=.75  heat_out=off  AC_pwr=on  pf=1  mech_pwr=off
  Left Wing Fuel Tank : PowerFlowLib/Energy & Power Systems/Thermal/Fuel/Fuel Tank  fileslct=off  filename=fueltank_area.m  filedir=C:\Users\mwillms4\Documents\My Box Files\Graduate\Research\PowerFlow Development\PowerFlow Fall 2013\SupportFunctions\fueltank_area.m  tank_loc=Left Wing Tank  areaprompt2=off  max_vol=3.2  m_init=2500  fld_Tint=0  ull_Tint=30  Pover=100  HTC_fg=14.2  wallHXF=off  wetHTC=14.2  dryHTC=14.2  Qinternal=0
  Pump Split : Subsystem
  Pump Split1 : Subsystem
  Pump Split2 : Subsystem
  Right Wing Fuel Pump #1 : PowerFlowLib/Energy & Power Systems/Thermal/Fuel/Fuel Pump  maptype=Pressure (kPa) vs. Vol. Flow Rate (m³/hr)  map=B737_AC_fuel1  map_load=off  SG=0.82  pump_eff=.75  heat_out=off  AC_pwr=on  pf=1  mech_pwr=off
  Right Wing Fuel Pump #2 : PowerFlowLib/Energy & Power Systems/Thermal/Fuel/Fuel Pump  maptype=Pressure (kPa) vs. Vol. Flow Rate (m³/hr)  map=B737_AC_fuel1  map_load=off  SG=0.82  pump_eff=.75  heat_out=off  AC_pwr=on  pf=1  mech_pwr=off
  Right Wing Fuel Tank : PowerFlowLib/Energy & Power Systems/Thermal/Fuel/Fuel Tank  fileslct=off  filename=fueltank_area.m  filedir=C:\Users\mwillms4\Documents\My Box Files\Graduate\Research\PowerFlow Development\PowerFlow Fall 2013\SupportFunctions\fueltank_area.m  tank_loc=Right Wing Tank  areaprompt2=off  max_vol=3.2  m_init=2500  fld_Tint=0  ull_Tint=30  Pover=100  HTC_fg=14.2  wallHXF=off  wetHTC=14.2  dryHTC=14.2  Qinternal=0
  Scope{,1..5} (6 alike) : Scope
      Scope settings: SaveName=ScopeData21
      Scope1 settings: YMin=2498.9  YMax=2498.9  SaveName=ScopeData23
      Scope2 settings: SaveName=ScopeData25
      Scope3 settings: SaveName=ScopeData27
      Scope4 settings: SaveName=ScopeData28
      Scope5 settings: SaveName=ScopeData29
  Terminator{,1..5} (6 alike) : Terminator
  Fuel Left Wing : Outport
  Fuel Right Wing : Outport  Port=2
  wires:
  Left  Wing Fuel Pump #2/3 -> Add6/2
  Left  Wing Fuel Pump #1/3 -> Add6/1
  Center Fuel Pump #2/3 -> Add4/2
  Center Fuel Pump #1/3 -> Add4/1
  Right Wing Fuel Pump #2/3 -> Add3/2
  Right Wing Fuel Pump #1/3 -> Add3/1
  Bus Selector10/2 -> ElectricalSink6/2  "<react_pwr_VAr>"
  Bus Selector10/1 -> ElectricalSink6/1  "<real_pwr_W>"
  Bus Selector9/2 -> ElectricalSink5/2  "<react_pwr_VAr>"
  Bus Selector9/1 -> ElectricalSink5/1  "<real_pwr_W>"
  Bus Selector7/2 -> ElectricalSink4/2  "<react_pwr_VAr>"
  Bus Selector7/1 -> ElectricalSink4/1  "<real_pwr_W>"
  Bus Selector6/2 -> ElectricalSink3/2  "<react_pwr_VAr>"
  Bus Selector6/1 -> ElectricalSink3/1  "<real_pwr_W>"
  Bus Selector4/2 -> ElectricalSink2/2  "<react_pwr_VAr>"
  Bus Selector4/1 -> ElectricalSink2/1  "<real_pwr_W>"
  Bus Selector2/2 -> ElectricalSink1/2  "<react_pwr_VAr>"
  Right Wing Fuel Pump #1/2 -> Bus Selector2/1
  Add3/1 -> [heat_tank_rght]
  Add4/1 -> [heat_tank_cen]
  Bus Selector2/1 -> ElectricalSink1/1  "<real_pwr_W>"
  Bus Selector15/1 -> [Fuel_RWing]  "<FuelFlowNeed_kgps>"
  Fuel Demand Right Wing/1 -> Bus Selector15/1
  Bus Selector/1 -> [Fuel_LWing]  "<FuelFlowNeed_kgps>"
  Pump Split2/1(Flow Out) -> Left  Wing Fuel Pump #2/1, Left  Wing Fuel Pump #1/1
  Fuel Control Left Wing/1(Fuel2Engine) -> Fuel Left Wing/1
  "Fuel Control Right Wing "/1(Fuel2Engine) -> Fuel Right Wing/1
  "Fuel Control Right Wing "/2(Fuel2Tank) -> [rw_fuel_rtrn]
  Fuel Control Left Wing/2(Fuel2Tank) -> [lw_fuel_rtrn]
  [Fuel_LWing] -> Fuel Control Left Wing/1(FuelNeed)
  [Fuel_RWing] -> "Fuel Control Right Wing "/1(FuelNeed)
  Fuel Demand Left Wing/1 -> Bus Selector/1
  Ground2/1 -> Left Wing Fuel Tank/5
  Ground1/1 -> Center Fuel Tank/5
  Ground/1 -> Right Wing Fuel Tank/5
  Left Wing Fuel Tank/3 -> Terminator5/1
  Left Wing Fuel Tank/2 -> Terminator4/1
  Center Fuel Tank/3 -> Terminator3/1
  Center Fuel Tank/2 -> Scope2/1, Terminator2/1
  Right Wing Fuel Tank/3 -> Terminator1/1
  Right Wing Fuel Tank/2 -> Scope1/1, Terminator/1
  [Fuel_RWing] -> Scope/1, Flow Junction/1
  [Fuel_LWing] -> Flow Junction1/1
  [pres_rght] -> Right Wing Fuel Pump #1/3
  [pres_rght] -> Right Wing Fuel Pump #2/3
  [pres_rght] -> Center Fuel Pump #1/3
  [pres_lft] -> Center Fuel Pump #2/3
  [pres_lft] -> Left  Wing Fuel Pump #2/3
  [pres_lft] -> Left  Wing Fuel Pump #1/3
  Bus Selector14/1 -> [pres_lft]  "<pres_kPa>"
  [lw_rpm] -> Left  Wing Fuel Pump #2/2
  [lw_rpm] -> Left  Wing Fuel Pump #1/2
  [cen_rpm] -> Center Fuel Pump #2/2
  [cen_rpm] -> Center Fuel Pump #1/2
  [rw_rpm] -> Right Wing Fuel Pump #2/2
  Bus Selector13/1 -> [pres_rght]  "<pres_kPa>"
  [heat_tank_rght] -> Right Wing Fuel Tank/4
  [heat_tank_cen] -> Center Fuel Tank/4
  [heat_tank_lft] -> Left Wing Fuel Tank/4
  Add6/1 -> [heat_tank_lft]
  [Pres_Amb_kPa] -> Left Wing Fuel Tank/3
  [Pres_Amb_kPa] -> Center Fuel Tank/3
  [Pres_Amb_kPa] -> Right Wing Fuel Tank/3
  Add2/1 -> [mdot_tank_cen]  "mdot_kgps"
  Bus Selector11/1 -> Add2/1  "<mdot_kgps>"
  Bus Selector12/1 -> Add2/2  "<mdot_kgps>"
  Add1/1 -> [mdot_tank_lft]  "mdot_kgps"
  Bus Selector1/1 -> Add1/1  "<mdot_kgps>"
  Bus Selector3/1 -> Add1/2  "<mdot_kgps>"
  Add5/1 -> [mdot_tank_rght]  "mdot_kgps"
  Bus Selector5/1 -> Add5/1  "<mdot_kgps>"
  Left Wing Fuel Tank/1 -> Pump Split2/1(Flow In)
  Pump Split/1(Flow Out) -> Center Fuel Pump #2/1, Center Fuel Pump #1/1
  [mdot_tank_lft] -> Left Wing Fuel Tank/2
  [mdot_tank_cen] -> Center Fuel Tank/2
  [mdot_tank_rght] -> Right Wing Fuel Tank/2
  Bus Selector8/1 -> Add5/2  "<mdot_kgps>"
  Pump Split1/1(Flow Out) -> Right Wing Fuel Pump #2/1, Right Wing Fuel Pump #1/1
  Right Wing Fuel Tank/1 -> Pump Split1/1(Flow In)
  [rw_rpm] -> Right Wing Fuel Pump #1/2
  Right Wing Fuel Pump #1/1 -> Scope3/1, Flow Junction/2, Bus Selector5/1
  Right Wing Fuel Pump #2/2 -> Bus Selector4/1
  [rw_fuel_rtrn] -> Right Wing Fuel Tank/1
  Right Wing Fuel Pump #2/1 -> Scope4/1, Flow Junction/3, Bus Selector8/1
  Center Fuel Tank/1 -> Pump Split/1(Flow In)
  Flow Junction/1 -> "Fuel Control Right Wing "/2(FuelFromPump), Bus Selector13/1  "to right wing engine"
  Center Fuel Pump #1/2 -> Bus Selector6/1
  Center Fuel Pump #1/1 -> Scope5/1, Flow Junction/4, Bus Selector11/1
  Flow Junction1/1 -> Fuel Control Left Wing/2(FuelFromPump), Bus Selector14/1  "to left wing engine"
  Center Fuel Pump #2/2 -> Bus Selector7/1
  FlowGenerator1/1(FlowOut) -> Center Fuel Tank/1
  Center Fuel Pump #2/1 -> Flow Junction1/2, Bus Selector12/1
  Left  Wing Fuel Pump #1/2 -> Bus Selector9/1
  Left  Wing Fuel Pump #1/1 -> Flow Junction1/3, Bus Selector1/1
  Left  Wing Fuel Pump #2/2 -> Bus Selector10/1
  [lw_fuel_rtrn] -> Left Wing Fuel Tank/1
  Left  Wing Fuel Pump #2/1 -> Flow Junction1/4, Bus Selector3/1
  Fuel Switch On/Off/3(Center RPM) -> [cen_rpm]
  Fuel Switch On/Off/2(Left Wing RPM) -> [lw_rpm]
  Fuel Switch On/Off/1(Right Wing RPM) -> [rw_rpm]
  Fuel Switch2/1 -> Fuel Switch On/Off/3(Left Wing Tank)
  Fuel Switch1/1 -> Fuel Switch On/Off/2(Center Tank)
  Fuel Switch/1 -> Fuel Switch On/Off/1(Right Wing Tank)
  Pamb/1 -> [Pres_Amb_kPa]

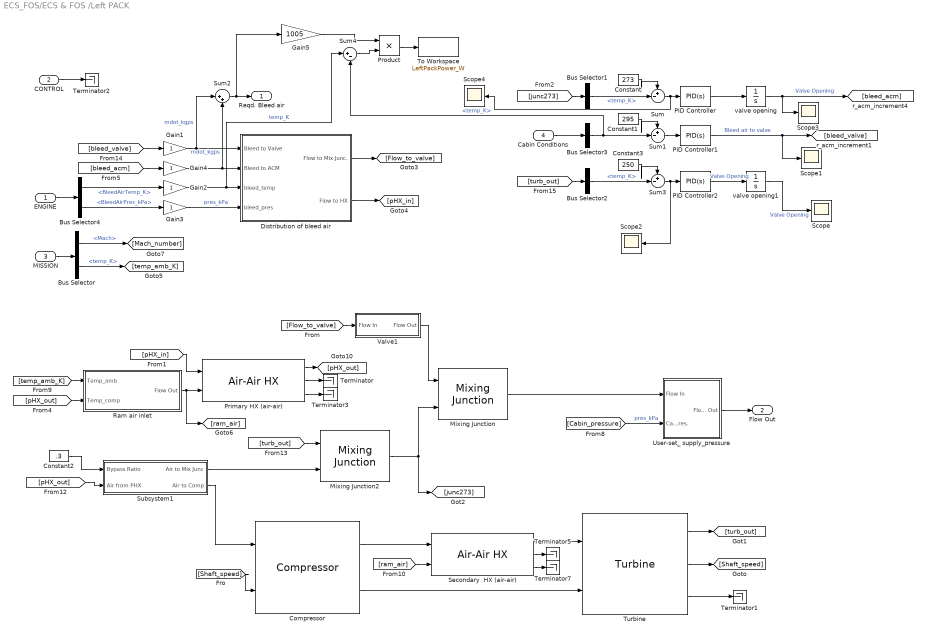
== system ECS_FOS/ECS & FOS /Left PACK ==
  ENGINE : Inport
  CONTROL : Inport  Port=2
  MISSION : Inport  Port=3
  Cabin Conditions : Inport  Port=4
  Bus Selector : BusSelector  OutputSignals=Flight parameters.Mach,Flight parameters.temp_K
  Bus Selector1 : BusSelector  OutputSignals=temp_K
  Bus Selector2 : BusSelector  OutputSignals=temp_K
  Bus Selector3 : BusSelector  OutputSignals=temp_K
  Bus Selector4 : BusSelector  OutputSignals=Bleed.BleedAirTemp_K,Bleed.BleedAirPres_kPa
  Compressor : PowerFlowLib/Energy & Power Systems/Thermal/ECS/Compressor
  Constant : Constant  Value=273
  Constant1 : Constant  Value=295
  Constant2 : Constant  Value=.3
  Constant3 : Constant  Value=250
  Distribution of bleed air : Subsystem
      mask Display:
      | port_label('input',1,'{ \bfBleed air to valve [kg/s]}','texmode','on')
      | port_label('input',2,'{ \bfBleed air to ACM [kg/s]}','texmode','on')
      | port_label('input',3,'{ \bfBleed temp. (K)}','texmode','on');
      | port_label('input',4,'{ \bfBleed pressure. (kPa)}','texmode','on')
      | 
      | 
      | 
      | port_label('output',1,'{\bfFlow to Mix Junc. }','texmode','on')
      | port_label('output',2,'{\bfFlow to ACM }','texmode','on')
  Gain{1..4} (4 alike) : Gain
  Gain5 : Gain  Gain=1005
  Mixing Junction : PowerFlowLib/Energy & Power Systems/Thermal/ECS/Mixing Junction  d_in_1=0.1  d_in_2=0.1  d_out=0.2
  Mixing Junction2 : PowerFlowLib/Energy & Power Systems/Thermal/ECS/Mixing Junction  d_in_1=0.1  d_in_2=0.1  d_out=0.2
  PID Controller : simulink/Continuous/PID Controller  Controller=PID  TimeDomain=Continuous-time  SampleTime=1  IntegratorMethod=Forward Euler  FilterMethod=Forward Euler  Form=Parallel  P=.01  I=0  D=0  N=100  InitialConditionSource=internal  InitialConditionForIntegrator=0  InitialConditionForFilter=0  ExternalReset=none  LimitOutput=off  UpperSaturationLimit=inf  LowerSaturationLimit=-inf  LinearizeAsGain=off  AntiWindupMode=none  Kb=1  TrackingMode=off  Kt=1  PParamMin=[]  PParamMax=[]  IParamMin=[]  IParamMax=[]  DParamMin=[]  DParamMax=[]  NParamMin=[]  NParamMax=[]  KbParamMin=[]  KbParamMax=[]  KtParamMin=[]  KtParamMax=[]  POutMin=[]  POutMax=[]  IOutMin=[]  IOutMax=[]  DOutMin=[]  DOutMax=[]  NOutMin=[]  NOutMax=[]  KbOutMin=[]  KbOutMax=[]  KtOutMin=[]  KtOutMax=[]  IntegratorOutMin=[]  IntegratorOutMax=[]  FilterOutMin=[]  FilterOutMax=[]  SumOutMin=[]  SumOutMax=[]  SumI1OutMin=[]  SumI1OutMax=[]  SumI2OutMin=[]  SumI2OutMax=[]  SumI3OutMin=[]  SumI3OutMax=[]  SumDOutMin=[]  SumDOutMax=[]  SaturationOutMin=[]  SaturationOutMax=[]  IntegratorContinuousStateAttributes=''  IntegratorStateMustResolveToSignalObject=off  IntegratorRTWStateStorageClass=Auto  FilterContinuousStateAttributes=''  FilterStateMustResolveToSignalObject=off  FilterRTWStateStorageClass=Auto
  PID Controller1 : simulink/Continuous/PID Controller  Controller=PID  TimeDomain=Continuous-time  SampleTime=1  IntegratorMethod=Forward Euler  FilterMethod=Forward Euler  Form=Parallel  P=.2  I=.01  D=0  N=100  InitialConditionSource=internal  InitialConditionForIntegrator=0  InitialConditionForFilter=0  ExternalReset=none  LimitOutput=on  UpperSaturationLimit=2  LowerSaturationLimit=.05  LinearizeAsGain=off  AntiWindupMode=none  Kb=1  TrackingMode=off  Kt=1  PParamMin=[]  PParamMax=[]  IParamMin=[]  IParamMax=[]  DParamMin=[]  DParamMax=[]  NParamMin=[]  NParamMax=[]  KbParamMin=[]  KbParamMax=[]  KtParamMin=[]  KtParamMax=[]  POutMin=[]  POutMax=[]  IOutMin=[]  IOutMax=[]  DOutMin=[]  DOutMax=[]  NOutMin=[]  NOutMax=[]  KbOutMin=[]  KbOutMax=[]  KtOutMin=[]  KtOutMax=[]  IntegratorOutMin=[]  IntegratorOutMax=[]  FilterOutMin=[]  FilterOutMax=[]  SumOutMin=[]  SumOutMax=[]  SumI1OutMin=[]  SumI1OutMax=[]  SumI2OutMin=[]  SumI2OutMax=[]  SumI3OutMin=[]  SumI3OutMax=[]  SumDOutMin=[]  SumDOutMax=[]  SaturationOutMin=[]  SaturationOutMax=[]  IntegratorContinuousStateAttributes=''  IntegratorStateMustResolveToSignalObject=off  IntegratorRTWStateStorageClass=Auto  FilterContinuousStateAttributes=''  FilterStateMustResolveToSignalObject=off  FilterRTWStateStorageClass=Auto
  PID Controller2 : simulink/Continuous/PID Controller  Controller=PID  TimeDomain=Continuous-time  SampleTime=1  IntegratorMethod=Forward Euler  FilterMethod=Forward Euler  Form=Parallel  P=0.01  I=0  D=0  N=100  InitialConditionSource=internal  InitialConditionForIntegrator=0  InitialConditionForFilter=0  ExternalReset=none  LimitOutput=off  UpperSaturationLimit=inf  LowerSaturationLimit=0  LinearizeAsGain=off  AntiWindupMode=none  Kb=1  TrackingMode=off  Kt=1  PParamMin=[]  PParamMax=[]  IParamMin=[]  IParamMax=[]  DParamMin=[]  DParamMax=[]  NParamMin=[]  NParamMax=[]  KbParamMin=[]  KbParamMax=[]  KtParamMin=[]  KtParamMax=[]  POutMin=[]  POutMax=[]  IOutMin=[]  IOutMax=[]  DOutMin=[]  DOutMax=[]  NOutMin=[]  NOutMax=[]  KbOutMin=[]  KbOutMax=[]  KtOutMin=[]  KtOutMax=[]  IntegratorOutMin=[]  IntegratorOutMax=[]  FilterOutMin=[]  FilterOutMax=[]  SumOutMin=[]  SumOutMax=[]  SumI1OutMin=[]  SumI1OutMax=[]  SumI2OutMin=[]  SumI2OutMax=[]  SumI3OutMin=[]  SumI3OutMax=[]  SumDOutMin=[]  SumDOutMax=[]  SaturationOutMin=[]  SaturationOutMax=[]  IntegratorContinuousStateAttributes=''  IntegratorStateMustResolveToSignalObject=off  IntegratorRTWStateStorageClass=Auto  FilterContinuousStateAttributes=''  FilterStateMustResolveToSignalObject=off  FilterRTWStateStorageClass=Auto
  Primary HX (air-air) : PowerFlowLib/Energy & Power Systems/Thermal/ECS/Air-Air HX  L_hx=0.2  W_hx=0.2  H_hx=0.2  t_p=0.0008  K_p=167  cp_hx=883  m_cm=16  l_fin=.005  t_fin=0.0002  s_fin=0.0015  h_fin=0.0095  K_n=167  eta_f=0.8  T_cm_0=50
  Product : Product
  Ram air inlet : Subsystem  mask{ram_air=.5, T_35=273}
      mask prompts: ram_air "Ram air mass flow rate"; T_35 "Temperature control for 35F valve"
      mask Display:
      | port_label('input',1,'{ \bf Ambient Temp.}','texmode','on')
      | port_label('input',2,'{ \bf Comp. Face Temp.}','texmode','on');
      | 
      | port_label('output',1,'{\bf Flow Out}','texmode','on')
  Scope{,1..4} (5 alike) : Scope
      Scope settings: YMin=0  YMax=1  SaveName=ScopeData32  SampleInput=on  SampleTime=1
      Scope1 settings: SaveName=ScopeData33  SampleInput=on  SampleTime=1
      Scope2 settings: YMin=-0.0534  YMax=-0.0529  SaveName=ScopeData34  SampleInput=on  SampleTime=1
      Scope3 settings: YMin=0.28294  YMax=0.28294  SaveName=ScopeData35  SampleInput=on  SampleTime=1
      Scope4 settings: TimeRange=1500  YMin=2.8421709427e-013  YMax=2.8421709434e-013  SaveName=ScopeData37  SampleInput=on  SampleTime=1
  Secondary  HX (air-air) : PowerFlowLib/Energy & Power Systems/Thermal/ECS/Air-Air HX  L_hx=0.2  W_hx=0.2  H_hx=0.2  t_p=0.0008  K_p=167  cp_hx=883  m_cm=16  l_fin=.005  t_fin=0.0002  s_fin=0.0015  h_fin=0.0095  K_n=167  eta_f=0.8  T_cm_0=25
  Subsystem1 : Subsystem
  Sum : Sum  Inputs=+-|
  Sum1 : Sum  Inputs=+-|
  Sum2 : Sum  Inputs=|++
  Sum3 : Sum  Inputs=+-|
  Sum4 : Sum  Inputs=|+-
  Terminator{,1..3,5,7} (6 alike) : Terminator
  To Workspace : ToWorkspace  VariableName=LeftPackPower_W  SampleTime=10  SaveFormat=Structure With Time
  Turbine : PowerFlowLib/Energy & Power Systems/Thermal/ECS/Turbine  press_Turbine_exit=80  inertia=5e-5  n_t=0.7
  User-set_ supply_pressure : Subsystem
  Valve1 : Subsystem
  valve opening : Integrator  InitialCondition=.4  LimitOutput=on  UpperSaturationLimit=.8  LowerSaturationLimit=.2
  valve opening1 : Integrator  InitialCondition=.5  LimitOutput=on  UpperSaturationLimit=1  LowerSaturationLimit=.3
  Reqd. Bleed air : Outport
  Flow Out : Outport  Port=2
  wires:
  Product/1 -> To Workspace/1
  Sum4/1 -> Product/2
  Gain5/1 -> Product/1
  Constant2/1 -> Subsystem1/1(Bypass Ratio)
  [bleed_acm] -> Gain4/1
  Cabin Conditions/1 -> Bus Selector3/1
  valve opening1/1 -> Scope/1  "Valve Opening"
  Constant3/1 -> Sum3/1
  PID Controller2/1 -> valve opening1/1  "Valve Opening"
  Sum3/1 -> Scope2/1, PID Controller2/1
  Bus Selector2/1 -> Sum3/2  "<temp_K>"
  [turb_out] -> Bus Selector2/1
  Sum2/1 -> Reqd. Bleed air/1, Gain5/1
  Gain4/1 -> Sum2/2, Distribution of bleed air/2(Bleed to ACM)  "mdot_kgps"
  Constant/1 -> Sum/1
  valve opening/1 -> [bleed_acm], Scope3/1  "Valve Opening"
  PID Controller/1 -> valve opening/1
  Sum/1 -> Scope4/1, PID Controller/1
  Bus Selector1/1 -> Sum/2  "<temp_K>"
  [junc273] -> Bus Selector1/1
  Subsystem1/2(Air to Comp) -> Compressor/1
  Subsystem1/1(Air to Mix Junc) -> Mixing Junction2/2
  [turb_out] -> Mixing Junction2/1
  Mixing Junction2/1 -> Mixing Junction/2, [junc273]
  [pHX_out] -> Subsystem1/2(Air from PHX)
  Secondary  HX (air-air)/1 -> Turbine/1
  Secondary  HX (air-air)/3 -> Terminator7/1
  Secondary  HX (air-air)/2 -> Terminator5/1
  Primary HX (air-air)/1 -> [pHX_out]
  Primary HX (air-air)/2 -> Terminator/1
  Primary HX (air-air)/3 -> Terminator3/1
  [bleed_valve] -> Gain1/1
  Gain3/1 -> Distribution of bleed air/4(bleed_pres)  "pres_kPa"
  Gain2/1 -> Distribution of bleed air/3(bleed_temp), Sum4/1  "temp_K"
  Gain1/1 -> Sum2/1, Distribution of bleed air/1(Bleed to Valve)  "mdot_kgps"
  Bus Selector/1 -> [Mach_number]  "<Mach>"
  Bus Selector/2 -> [temp_amb_K]  "<temp_K>"
  Bus Selector4/2 -> Gain3/1  "<BleedAirPres_kPa>"
  Bus Selector4/1 -> Gain2/1  "<BleedAirTemp_K>"
  Distribution of bleed air/1(Flow to Mix Junc.) -> [Flow_to_valve]
  Distribution of bleed air/2(Flow to HX) -> [pHX_in]
  ENGINE/1 -> Bus Selector4/1
  CONTROL/1 -> Terminator2/1
  MISSION/1 -> Bus Selector/1
  [pHX_out] -> Ram air inlet/2(Temp_comp)
  [temp_amb_K] -> Ram air inlet/1(Temp_amb)
  [Cabin_pressure] -> User-set_ supply_pressure/2(Cabin Pres.)  "pres_kPa"
  User-set_ supply_pressure/1(Flow Out) -> Flow Out/1
  Turbine/1 -> [turb_out]
  Turbine/3 -> Terminator1/1
  Turbine/2 -> [Shaft_speed]
  Mixing Junction/1 -> User-set_ supply_pressure/1(Flow In)
  [ram_air] -> Secondary  HX (air-air)/2
  Compressor/1 -> Secondary  HX (air-air)/1
  Ram air inlet/1(Flow Out) -> [ram_air], Primary HX (air-air)/2
  Compressor/2 -> Turbine/2
  [Shaft_speed] -> Compressor/2
  [Flow_to_valve] -> Valve1/1(Flow In)
  Valve1/1(Flow Out) -> Mixing Junction/1
  [pHX_in] -> Primary HX (air-air)/1
  Bus Selector3/1 -> Sum1/2, Sum4/2  "<temp_K>"
  Sum1/1 -> PID Controller1/1
  PID Controller1/1 -> Scope1/1, [bleed_valve]  "Bleed air to valve"
  Constant1/1 -> Sum1/1

== system ECS_FOS/ECS & FOS /Oil Tanks//Pumps Left Wing ==
  Oil Sys Pres : Inport
  Flow In : Inport  Port=2
  Bus Selector1 : BusSelector  OutputSignals=Oil
  Bus Selector2 : BusSelector  OutputSignals=real_pwr_W,react_pwr_VAr
  Bus Selector5 : BusSelector  OutputSignals=mdot_kgps,pres_kPa
  ElectricalSink1 : PowerFlowLib/Support Functions//Tools/ElectricalSink  Tag=Flow  Description=TwoPhase  load_loc=LeftWing  ACDC_load=AC  units=Watts  unq_id=9405
  Fuel Switch2 : Constant  Value=1400
  Ground : Ground
  Ground1 : Ground
  Oil Pump : PowerFlowLib/Energy & Power Systems/Thermal/Oil/Oil Pump  maptype=Pressure (kPa) vs. Vol. Flow Rate (m³/hr)  map=B737_mech_fuel1  map_load=off  SG=0.82  pump_eff=.75  heat_out=off  AC_pwr=on  pf=1  mech_pwr=off
  Oil Tank : PowerFlowLib/Energy & Power Systems/Thermal/Fuel/Fuel Tank  fileslct=off  filename=fueltank_area.m  filedir=C:\Users\mwillms4\Documents\My Box Files\Graduate\Research\PowerFlow Development\PowerFlow Fall 2013\SupportFunctions\fueltank_area.m  tank_loc=Left Wing Tank  areaprompt2=off  max_vol=3.2  m_init=2500  fld_Tint=0  ull_Tint=30  Pover=100  HTC_fg=14.2  wallHXF=off  wetHTC=14.2  dryHTC=14.2  Qinternal=0
  Terminator : Terminator
  Terminator1 : Terminator
  Oil To HX : Outport
  wires:
  Bus Selector1/1 -> Oil Tank/1  "<Oil>"
  Oil Pump/2 -> Bus Selector2/1
  Bus Selector2/2 -> ElectricalSink1/2  "<react_pwr_VAr>"
  Bus Selector2/1 -> ElectricalSink1/1  "<real_pwr_W>"
  Oil Tank/1 -> Oil Pump/1
  Oil Tank/2 -> Terminator/1
  Oil Tank/3 -> Terminator1/1
  Ground/1 -> Oil Tank/5
  Oil Pump/3 -> Oil Tank/4
  Oil Pump/1 -> Bus Selector5/1, Oil To HX/1
  Ground1/1 -> Oil Tank/3
  Oil Sys Pres/1 -> Oil Pump/3
  Flow In/1 -> Bus Selector1/1
  Fuel Switch2/1 -> Oil Pump/2
  Bus Selector5/1 -> Oil Tank/2  "<mdot_kgps>"

== system ECS_FOS/ECS & FOS /Oil Tanks//Pumps Right Wing ==
  Oil Sys Pres : Inport
  Flow In : Inport  Port=2
  Bus Selector1 : BusSelector  OutputSignals=Oil
  Bus Selector2 : BusSelector  OutputSignals=real_pwr_W,react_pwr_VAr
  Bus Selector5 : BusSelector  OutputSignals=mdot_kgps,pres_kPa
  ElectricalSink1 : PowerFlowLib/Support Functions//Tools/ElectricalSink  Tag=Flow  Description=TwoPhase  load_loc=RightWing  ACDC_load=AC  units=Watts  unq_id=2169
  Fuel Switch2 : Constant  Value=1400
  Fuel Tank : PowerFlowLib/Energy & Power Systems/Thermal/Fuel/Fuel Tank  fileslct=off  filename=fueltank_area.m  filedir=C:\Users\mwillms4\Documents\My Box Files\Graduate\Research\PowerFlow Development\PowerFlow Fall 2013\SupportFunctions\fueltank_area.m  tank_loc=Left Wing Tank  areaprompt2=off  max_vol=3.2  m_init=2500  fld_Tint=0  ull_Tint=30  Pover=100  HTC_fg=14.2  wallHXF=off  wetHTC=14.2  dryHTC=14.2  Qinternal=0
  Ground : Ground
  Ground1 : Ground
  Oil Pump : PowerFlowLib/Energy & Power Systems/Thermal/Oil/Oil Pump  maptype=Pressure (kPa) vs. Vol. Flow Rate (m³/hr)  map=B737_mech_fuel1  map_load=off  SG=0.82  pump_eff=.75  heat_out=off  AC_pwr=on  pf=1  mech_pwr=off
  Terminator : Terminator
  Terminator1 : Terminator
  Oil To HX : Outport
  wires:
  Bus Selector1/1 -> Fuel Tank/1  "<Oil>"
  Oil Pump/2 -> Bus Selector2/1
  Bus Selector2/2 -> ElectricalSink1/2  "<react_pwr_VAr>"
  Bus Selector2/1 -> ElectricalSink1/1  "<real_pwr_W>"
  Bus Selector5/1 -> Fuel Tank/2  "<mdot_kgps>"
  Fuel Switch2/1 -> Oil Pump/2
  Flow In/1 -> Bus Selector1/1
  Oil Sys Pres/1 -> Oil Pump/3
  Ground1/1 -> Fuel Tank/3
  Oil Pump/1 -> Oil To HX/1, Bus Selector5/1
  Oil Pump/3 -> Fuel Tank/4
  Ground/1 -> Fuel Tank/5
  Fuel Tank/3 -> Terminator1/1
  Fuel Tank/2 -> Terminator/1
  Fuel Tank/1 -> Oil Pump/1
